simulink model "Phase_Shift_Keying"  (R2023b)
settings: Solver=VariableStepAuto  StartTime=0.0  StopTime=10.0  RelTol=1e-3
settings Model: Creator=online  LastModifiedBy=online

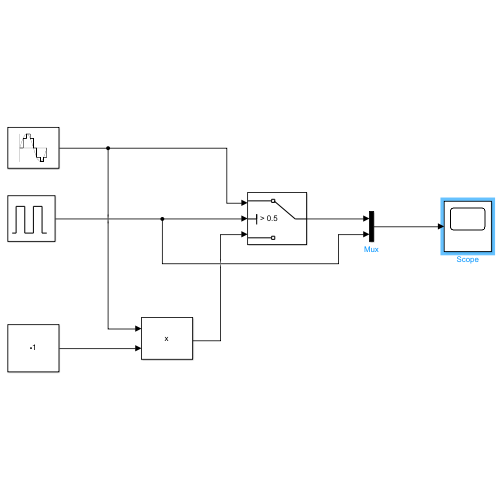
[thumbnail: Simulink's stored preview of the top-level diagram]
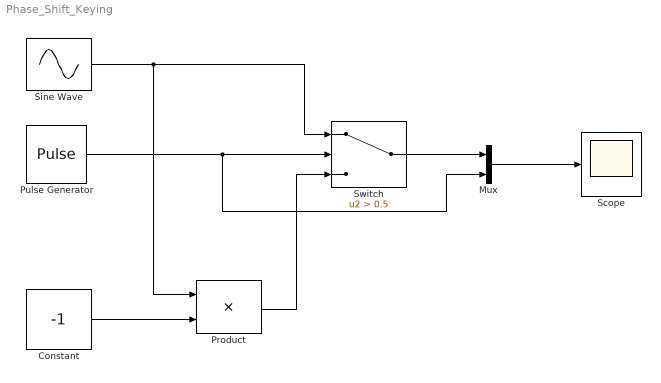
== system Phase_Shift_Keying ==
  Constant : Constant  Value=-1
  Mux : Mux  Inputs=2
  Product : Product
  Pulse Generator : DiscretePulseGenerator  PulseType=Time based  PulseWidth=50
  Scope : Scope
  Sine Wave : Sin  Frequency=2*pi*2  SampleTime=0.01
  Switch : Switch  Criteria=u2 > Threshold  Threshold=0.5  SaturateOnIntegerOverflow=off  InputSameDT=off
  wires:
  Constant/1 -> Product/2
  Sine Wave/1 -> Product/1, Switch/1
  Product/1 -> Switch/3
  Switch/1 -> Mux/1
  Mux/1 -> Scope/1
  Pulse Generator/1 -> Mux/2, Switch/2
